simulink model "Assignment1Final"  (R2020a)
settings: Solver=FixedStepAuto  StartTime=0.0  StopTime=10.0  FixedStep=1e-3  RelTol=1e-3  EnableMultiTasking=on
undefined symbols (not defined in the file): D0, D1, D10, D11, D12, D13, D2, D3, D4, D5, D6, D7, D8, D9, PTA0, PTA1, PTA2, PTB23, PTB9, PTC16, PTC17, PTC2, PTC3, PTC4, PTD0, PTD1, PTD2, PTD3
libraries: frdmk64flib x14
settings Model: ExtModeTrigDuration=5  Creator=mance  LastModifiedBy=mance
settings OptimizationCC: EnhancedBackFolding=on  PassReuseOutputArgsAs=Individual arguments  ZeroExternalMemoryAtStartup=off  ZeroInternalMemoryAtStartup=off  MaxStackSize=64  OptimizeBlockOrder=speed  DifferentSizesBufferReuse=on  OptimizationCustomize=off  EfficientTunableParamExpr=on
settings DebuggingCC: ParameterTunabilityLossMsg=error
settings HardwareCC: ProdBitPerPointer=32  ProdBitPerSizeT=32  ProdBitPerPtrDiffT=32  ProdLargestAtomicInteger=Long  ProdLargestAtomicFloat=Double  ProdWordSize=32  ProdHWDeviceType=ARM Compatible->ARM Cortex
settings SFSimCC: MATLABDynamicMemAlloc=off
settings RTWCC: SystemTargetFile=ert.tlc  HardwareBoard=NXP FRDM-K64F  TemplateMakefile=ert_default_tmf  Toolchain=GNU Tools for ARM Embedded Processors
settings CodeAppCC: ForceParamTrailComments=on  IgnoreCustomStorageClasses=off  OperatorAnnotations=on  SimulinkDataObjDesc=on  SFDataObjDesc=on  InsertBlockDesc=on

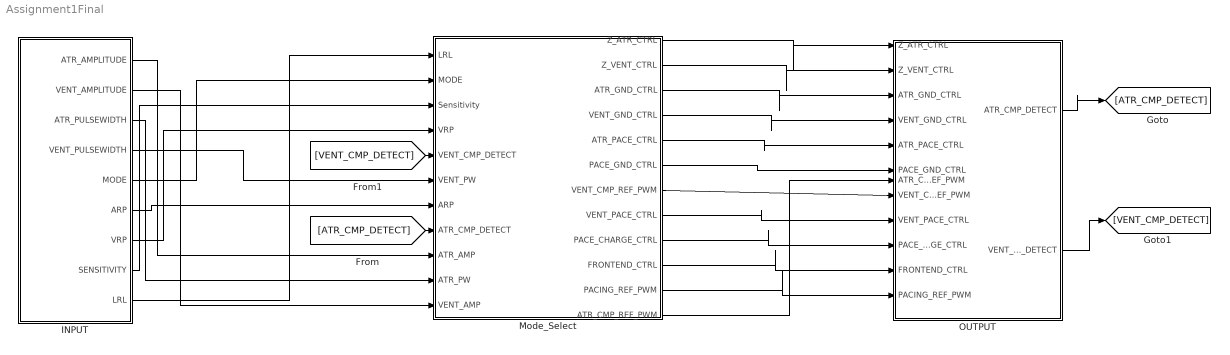
== system Assignment1Final ==
  INPUT : Subsystem
  Mode_Select : Stateflow chart  TreatAsAtomicUnit=on
  OUTPUT : Subsystem
  wires:
  Mode_Select/1(Z_ATR_CTRL) -> OUTPUT/1(Z_ATR_CTRL)
  Mode_Select/2(Z_VENT_CTRL) -> OUTPUT/2(Z_VENT_CTRL)
  Mode_Select/3(ATR_GND_CTRL) -> OUTPUT/3(ATR_GND_CTRL)
  Mode_Select/4(VENT_GND_CTRL) -> OUTPUT/4(VENT_GND_CTRL)
  Mode_Select/5(ATR_PACE_CTRL) -> OUTPUT/5(ATR_PACE_CTRL)
  Mode_Select/6(PACE_GND_CTRL) -> OUTPUT/6(PACE_GND_CTRL)
  Mode_Select/7(VENT_CMP_REF_PWM) -> OUTPUT/7(VENT_CMP_REF_PWM)
  Mode_Select/8(VENT_PACE_CTRL) -> OUTPUT/8(VENT_PACE_CTRL)
  Mode_Select/9(PACE_CHARGE_CTRL) -> OUTPUT/9(PACE_CHARGE_CTRL)
  Mode_Select/10(FRONTEND_CTRL) -> OUTPUT/10(FRONTEND_CTRL)
  Mode_Select/11(PACING_REF_PWM) -> OUTPUT/11(PACING_REF_PWM)
  Mode_Select/12(ATR_CMP_REF_PWM) -> OUTPUT/12(ATR_CMP_REF_PWM)
  OUTPUT/1(ATR_CMP_DETECT) -> [ATR_CMP_DETECT]
  OUTPUT/2(VENT_CMP_DETECT) -> [VENT_CMP_DETECT]
  [ATR_CMP_DETECT] -> Mode_Select/8(ATR_CMP_DETECT)
  [VENT_CMP_DETECT] -> Mode_Select/5(VENT_CMP_DETECT)
  INPUT/5(MODE) -> Mode_Select/2(MODE)
  INPUT/6(ARP) -> Mode_Select/7(ARP)
  INPUT/7(VRP) -> Mode_Select/4(VRP)
  INPUT/9(LRL) -> Mode_Select/1(LRL)
  INPUT/1(ATR_AMPLITUDE) -> Mode_Select/9(ATR_AMP)
  INPUT/2(VENT_AMPLITUDE) -> Mode_Select/11(VENT_AMP)
  INPUT/8(SENSITIVITY) -> Mode_Select/3(Sensitivity)
  INPUT/3(ATR_PULSEWIDTH) -> Mode_Select/10(ATR_PW)
  INPUT/4(VENT_PULSEWIDTH) -> Mode_Select/6(VENT_PW)

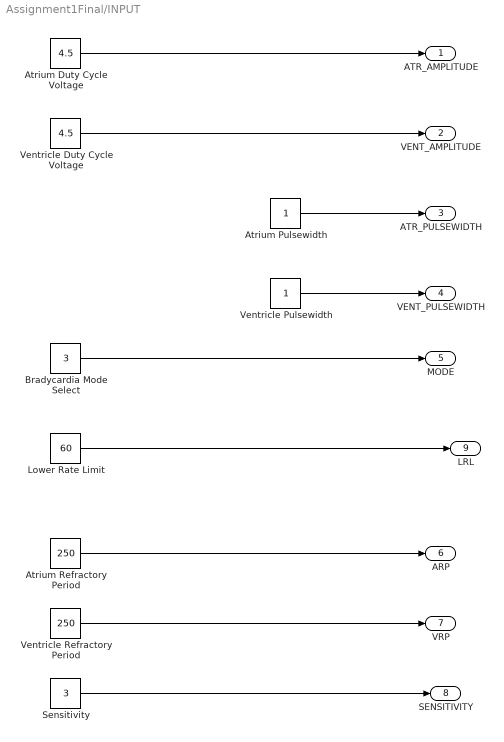
== system Assignment1Final/INPUT ==
  Atrium Duty Cycle Voltage : Constant  Value=4.5
  Atrium Pulsewidth : Constant
  Atrium Refractory Period : Constant  Value=250
  Bradycardia Mode Select : Constant  Value=3
  Lower Rate Limit : Constant  Value=60
  Sensitivity : Constant  Value=3
  Ventricle Duty Cycle Voltage : Constant  Value=4.5
  Ventricle Pulsewidth : Constant
  Ventricle Refractory Period : Constant  Value=250
  ATR_AMPLITUDE : Outport
  VENT_AMPLITUDE : Outport  Port=2
  ATR_PULSEWIDTH : Outport  Port=3
  VENT_PULSEWIDTH : Outport  Port=4
  MODE : Outport  Port=5
  ARP : Outport  Port=6
  VRP : Outport  Port=7
  SENSITIVITY : Outport  Port=8
  LRL : Outport  Port=9
  wires:
  Atrium Pulsewidth/1 -> ATR_PULSEWIDTH/1
  Sensitivity/1 -> SENSITIVITY/1
  Bradycardia Mode Select/1 -> MODE/1
  Ventricle Pulsewidth/1 -> VENT_PULSEWIDTH/1
  Ventricle Refractory Period/1 -> VRP/1
  Atrium Refractory Period/1 -> ARP/1
  Lower Rate Limit/1 -> LRL/1
  Atrium Duty Cycle Voltage/1 -> ATR_AMPLITUDE/1
  Ventricle Duty Cycle Voltage/1 -> VENT_AMPLITUDE/1

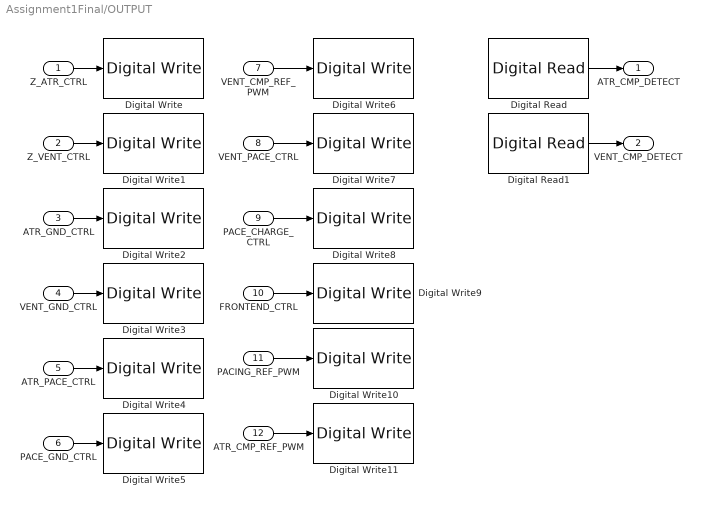
== system Assignment1Final/OUTPUT ==
  Z_ATR_CTRL : Inport
  Z_VENT_CTRL : Inport  Port=2
  ATR_GND_CTRL : Inport  Port=3
  VENT_GND_CTRL : Inport  Port=4
  ATR_PACE_CTRL : Inport  Port=5
  PACE_GND_CTRL : Inport  Port=6
  VENT_CMP_REF_PWM : Inport  Port=7
  VENT_PACE_CTRL : Inport  Port=8
  PACE_CHARGE_CTRL : Inport  Port=9
  FRONTEND_CTRL : Inport  Port=10
  PACING_REF_PWM : Inport  Port=11
  ATR_CMP_REF_PWM : Inport  Port=12
  Digital Read : frdmk64flib/Digital Read  Whichpin=PTC16 (D0)  SampleTime=-1
  Digital Read1 : frdmk64flib/Digital Read  Whichpin=PTC17 (D1)  SampleTime=-1
  Digital Write : frdmk64flib/Digital Write  Whichpin=PTB23 (D4)
  Digital Write1 : frdmk64flib/Digital Write  Whichpin=PTC3 (D7)
  Digital Write10 : frdmk64flib/Digital Write  Whichpin=PTA2 (D5)
  Digital Write11 : frdmk64flib/Digital Write  Whichpin=PTC2 (D6)
  Digital Write2 : frdmk64flib/Digital Write  Whichpin=PTD2 (D11)
  Digital Write3 : frdmk64flib/Digital Write  Whichpin=PTD3 (D12)
  Digital Write4 : frdmk64flib/Digital Write  Whichpin=PTA0 (D8)
  Digital Write5 : frdmk64flib/Digital Write  Whichpin=PTD0 (D10)
  Digital Write6 : frdmk64flib/Digital Write  Whichpin=PTA1 (D3)
  Digital Write7 : frdmk64flib/Digital Write  Whichpin=PTC4 (D9)
  Digital Write8 : frdmk64flib/Digital Write  Whichpin=PTB9 (D2)
  Digital Write9 : frdmk64flib/Digital Write  Whichpin=PTD1 (D13)
  ATR_CMP_DETECT : Outport
  VENT_CMP_DETECT : Outport  Port=2
  wires:
  Z_ATR_CTRL/1 -> Digital Write/1
  PACING_REF_PWM/1 -> Digital Write10/1
  ATR_GND_CTRL/1 -> Digital Write2/1
  Digital Read1/1 -> VENT_CMP_DETECT/1
  VENT_GND_CTRL/1 -> Digital Write3/1
  FRONTEND_CTRL/1 -> Digital Write9/1
  Digital Read/1 -> ATR_CMP_DETECT/1
  Z_VENT_CTRL/1 -> Digital Write1/1
  ATR_CMP_REF_PWM/1 -> Digital Write11/1
  PACE_GND_CTRL/1 -> Digital Write5/1
  VENT_CMP_REF_PWM/1 -> Digital Write6/1
  VENT_PACE_CTRL/1 -> Digital Write7/1
  PACE_CHARGE_CTRL/1 -> Digital Write8/1
  ATR_PACE_CTRL/1 -> Digital Write4/1

== stateflow chart Assignment1Final/Mode_Select ==
  state V_OO
    entry:
    %C22 closed meaning it charges
    ATR_PACE_CTRL = false
    VENT_PACE_CTRL = false
    PACING_REF_PWM = VENT_AMP*20
    PACE_CHARGE_CTRL = true
    %Discharging C21(blocking capacitor)
    PACE_GND_CTRL = true
    Z_ATR_CTRL = false
    Z_VENT_CTRL = false
    ATR_GND_CTRL = false
    VENT_GND_CTRL = true
  state V_OOpace
    entry:
    %Discharging C22 into AV to charge C21
    PACE_CHARGE_CTRL = false
    PACE_GND_CTRL = true
    ATR_PACE_CTRL = false
    ATR_GND_CTRL = false
    Z_ATR_CTRL = false
    Z_VENT_CTRL = false
    VENT_GND_CTRL = false
    VENT_PACE_CTRL = true
  note: VOO
  state MODE
    entry:
    VENT_GND_CTRL=false;
    Z_ATR_CTRL = false;
    Z_VENT_CTRL = false;
    FRONTEND_CTRL=false;
    PACE_CHARGE_CTRL = false;
    VENT_PACE_CTRL = false;
    ATR_PACE_CTRL = false;
    PACE_GND_CTRL=false;
    ATR_GND_CTRL=false;
  note: AOO
  state Pacing
    entry:
    PACE_CHARGE_CTRL = false;
    PACE_GND_CTRL = true;
    VENT_PACE_CTRL = false;
    VENT_GND_CTRL = false;
    Z_ATR_CTRL = false;
    Z_VENT_CTRL = false;
    ATR_GND_CTRL = false;
    ATR_PACE_CTRL = true;
  state Charging_C22_Discharging_C21
    entry:
    ATR_PACE_CTRL = false;
    VENT_PACE_CTRL = false;
    PACE_CHARGE_CTRL = true;
    PACE_GND_CTRL = true;
    Z_ATR_CTRL = false;
    Z_VENT_CTRL = false;
    ATR_GND_CTRL = true;
    VENT_GND_CTRL = false;
    PACING_REF_PWM = (ATR_AMP/5)*100
  state AAI_Charge_C22
    entry:
    ATR_PACE_CTRL = false;
    VENT_PACE_CTRL = false;
    PACING_REF_PWM = ATR_AMP * 20;
    PACE_CHARGE_CTRL = true;
    FRONTEND_CTRL = false;
    PACE_GND_CTRL = true;
    VENT_PACE_CTRL = false;
    ATR_GND_CTRL = true;
    VENT_GND_CTRL = false;
    PaceCycle = (60000/LRL) - ARP - ATR_PW;
  state AAI_Pace
    entry:
    PACE_CHARGE_CTRL = false;
    PACE_GND_CTRL = true;
    ATR_GND_CTRL = false;
    ATR_PACE_CTRL = true;
    VENT_PACE_CTRL = false;
    VENT_GND_CTRL = false;
    FRONTEND_CTRL = true;
    PACING_REF_PWM = ATR_AMP*20
    PaceCycle = (60000/LRL) - ARP - ATR_PW;
  note: AAI
  state AAI_Sense
    entry:
    PACE_CHARGE_CTRL = true;
    PACE_GND_CTRL = true;
    ATR_GND_CTRL = true;
    ATR_PACE_CTRL = false;
    FRONTEND_CTRL = true;
    PACING_REF_PWM = ATR_AMP*20;
    ATR_CMP_REF_PWM = (Sensitivity)*20
  state VVI_Charge
    entry:
    % Charges primary capacitor
    ATR_PACE_CTRL = false;
    VENT_PACE_CTRL = false;
    PACING_REF_PWM = VENT_AMP * 20;
    PACE_CHARGE_CTRL = true;
    FRONTEND_CTRL = false;
    % Discharging blocking capacitor
    PACE_GND_CTRL = true;
    VENT_PACE_CTRL = false;
    ATR_PACE_CTRL = false;
    ATR_GND_CTRL = false;
    VENT_GND_CTRL = true;
  state VVI_Pace
    entry:
    % Paces ventricle
    PACE_CHARGE_CTRL = false;
    PACE_GND_CTRL = true;
    ATR_PACE_CTRL = false;
    ATR_GND_CTRL = false;
    VENT_GND_CTRL = false;
    VENT_PACE_CTRL = true;
    FRONTEND_CTRL = true;
    PACING_REF_PWM = VENT_AMP * 20;
  note: VVI
  state VVI_Sense
    entry:
    PACE_CHARGE_CTRL = true;
    PACE_GND_CTRL = true;
    VENT_GND_CTRL = true;
    VENT_PACE_CTRL = false;
    FRONTEND_CTRL = true;
    PACING_REF_PWM = VENT_AMP * 20;
    VENT_CMP_REF_PWM = (Sensitivity)*20;
  V_OOpace -> V_OO : after(VENT_PW, msec)
  MODE -> V_OO [order 1] : [MODE==1]
  V_OO -> V_OOpace : after(((60000/LRL)-VENT_PW),msec)
  (default) -> MODE
  MODE -> Charging_C22_Discharging_C21 [order 2] : [MODE ==2]
  Charging_C22_Discharging_C21 -> Pacing : [after(60000/LRL-ATR_PW,msec)]
  MODE -> AAI_Charge_C22 [order 3] : [MODE ==3]
  Pacing -> Charging_C22_Discharging_C21 : [after(ATR_PW,msec)]
  MODE -> VVI_Charge [order 4] : [MODE == 4]
  AAI_Charge_C22 -> AAI_Pace [order 2] : after(PaceCycle, msec)
  AAI_Sense -> AAI_Charge_C22 : after(ARP, msec)
  AAI_Pace -> AAI_Sense : after(ATR_PW, msec)
  AAI_Charge_C22 -> AAI_Sense [order 1] : [ATR_CMP_DETECT == true]
      | {PaceCycle = ((60000/LRL) - ARP)}
  VVI_Charge -> VVI_Pace [order 2] : after((60000/LRL) - VRP - VENT_PW, msec)
  VVI_Pace -> VVI_Sense : after(VENT_PW, msec)
  VVI_Sense -> VVI_Charge : after(VRP, msec)
  VVI_Charge -> VVI_Sense [order 1] : [VENT_CMP_DETECT == true]{(60000/LRL) - VRP}
  data: Z_ATR_CTRL output; Z_VENT_CTRL output; ATR_GND_CTRL output; VENT_GND_CTRL output; ATR_PACE_CTRL output; LRL input; MODE input; Sensitivity input; VRP input; VENT_CMP_DETECT input; PACE_GND_CTRL output; VENT_CMP_REF_PWM output; VENT_PACE_CTRL output; PACE_CHARGE_CTRL output; FRONTEND_CTRL output; PACING_REF_PWM output; VENT_PW input; ATR_CMP_REF_PWM output; ARP input; ATR_CMP_DETECT input; PaceCycle local; ATR_AMP input; ATR_PW input; VENT_AMP input
